simulink model "untitled2"  (R2024a)
settings: Solver=VariableStepAuto  StartTime=0.0  StopTime=200  RelTol=1e-3
settings Model: Creator=Leti  LastModifiedBy=Leti

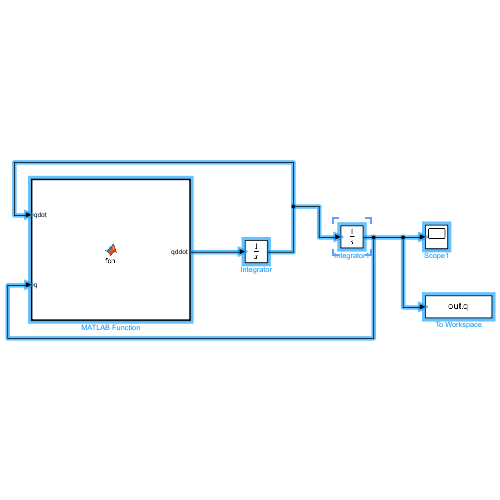
[thumbnail: Simulink's stored preview of the top-level diagram]
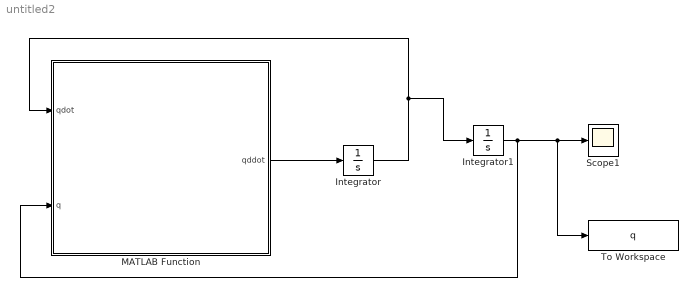
== system untitled2 ==
  Integrator : Integrator  InitialCondition=[0;0]
  Integrator1 : Integrator  InitialCondition=[-0.051558;-0.09618]
  MATLAB Function : MATLAB Function  TreatAsAtomicUnit=on
  Scope1 : Scope
  To Workspace : ToWorkspace  VariableName=q  SampleTime=-1
  wires:
  Integrator1/1 -> Scope1/1, To Workspace/1, MATLAB Function/2(q)
  MATLAB Function/1(qddot) -> Integrator/1
  Integrator/1 -> MATLAB Function/1(qdot), Integrator1/1

== matlab function untitled2/MATLAB Function ==
  data: qdot input; q input; qddot output


function qddot = fcn(qdot,q)


% Variables

g = 9.81;
Lp = 0.5;
Lw = 1;
Mp = 1;
Mw = 0.2;
Jp = 0.083;
Jw = 0.1;
dphi = 0;
ktheta = 6.558;
dtheta = 0;
theta_ref = pi/2;
kphi = 0.114;
phi_ref = pi/2;


q1 = [q(1)-1.04762 ; q(2)-pi/2];


% Matrices

M = [Mp*Lp^2 + Mw*Lw^2 + Jp + Jw , Jw ; Jw , Jw];

D = [dtheta , 0 ; 0 , dphi];

K = [ktheta - 0.5*sqrt(3)*g*(Lp*Mp + Lw*Mw) , 0 ; 0 , kphi];

Kt = [0,0;0,0];

Ktot = K+Kt;

Qt = [0;0];

    
% Motion

qddot = (M \ (Qt - D * qdot - Ktot * q1));
